simulink model "simulink_caso1_adc"  (R2023a)
settings: Solver=VariableStepAuto  StartTime=0.0  StopTime=10.0  RelTol=1e-3
undefined symbols (not defined in the file): A, Aestd, B, Bestd, C, Cestd, D, Destd, K0d, Kd, TS, X0
settings Model: Creator=Agustin  LastModifiedBy=Agustin

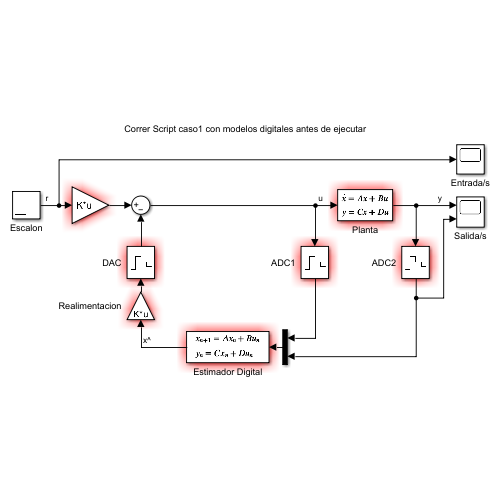
[thumbnail: Simulink's stored preview of the top-level diagram]
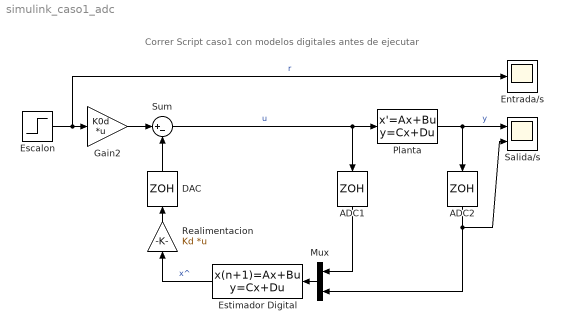
== system simulink_caso1_adc ==
  note: Correr Script caso1 con modelos digitales antes de ejecutar
  ADC1 : ZeroOrderHold  SampleTime=TS
  ADC2 : ZeroOrderHold  SampleTime=TS
  DAC : ZeroOrderHold  SampleTime=TS
  Entrada/s : Scope
  Escalon : Step  SampleTime=0
  Estimador Digital : DiscreteStateSpace  A=Aestd  B=Bestd  C=Cestd  D=Destd  SampleTime=TS
  Gain2 : Gain  Gain=K0d  Multiplication=Matrix(K*u)
  Mux : Mux  Inputs=2
  Planta : StateSpace  A=A  B=B  C=C  D=D  InitialCondition=X0
  Realimentacion : Gain  Gain=Kd  Multiplication=Matrix(K*u)
  Salida/s : Scope  NumInputPorts=2
  Sum : Sum  Inputs=|+-
  wires:
  Estimador Digital/1 -> Realimentacion/1  "x^"
  Sum/1 -> Planta/1, ADC1/1  "u"
  Planta/1 -> Salida/s/1, ADC2/1  "y"
  Escalon/1 -> Entrada/s/1, Gain2/1  "r"
  Mux/1 -> Estimador Digital/1
  Realimentacion/1 -> DAC/1
  Gain2/1 -> Sum/1
  DAC/1 -> Sum/2
  ADC1/1 -> Mux/1
  ADC2/1 -> Salida/s/2, Mux/2
